simulink model "LQR_c_2017a"  (R2017a)
settings: Solver=VariableStepAuto  StartTime=0.0  StopTime=30  RelTol=1e-3
values from neighbouring files (symbols this model uses):
  LQRopt = lqrd(A,B,Q,R,8e-5)    [initParams.m]    (also in teste.m)
settings Model: Creator=seumagal  LastModifiedBy=seumagal

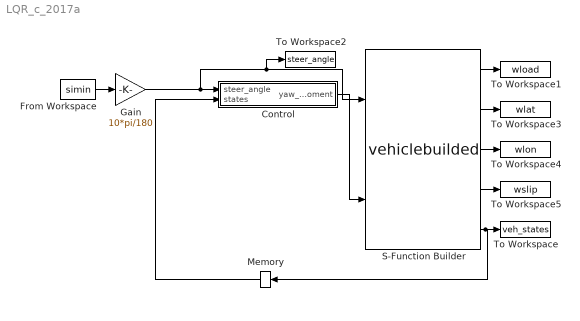
== system LQR_c_2017a ==
  "Control " : Subsystem  TreatAsAtomicUnit=on
  From Workspace : FromWorkspace  VariableName=simin  SampleTime=0
  Gain : Gain  Gain=10*pi/180
  Memory : Memory
  S-Function Builder : S-Function  InitFcn=try, set_param(gcb,'FunctionName','vehiclebuilded'), end  FunctionName=vehiclebuilded  Parameters=params  SFunctionModules=vehiclebuilded_wrapper  SFunctionDeploymentMode=off  EnableBusSupport=off  mask(S-Function Builder){}
      mask help: Simulink:masks:SFunctionBuilder_MD
      mask init:
      | val = [[.9  0.75 0.75 1 1 .9 .9 1]',[1 1 0.75 0.75 .9 .9 1 .9]'];try , sys = get_param(gcb,'SfunBuilderFcnName');if isempty(sys), sys = get_param(gcb,'FunctionName'); end,catch, sys = get_param(gcb,'FunctionName'); end
      settings: CopyFcn=set_param(gcbh,'LinkStatus','none')  PreSaveFcn=try, set_param(gcb,'FunctionName','vehiclebuilded'), end  OpenFcn=sfunctionwizard(gcbh)
      mask Display:
      | plot(val(:,1),val(:,2))
      | disp(sys)
      | port_label('input',1,'inSteer')
      | port_label('input',2,'inMz')
      | port_label('output',1,'outFz')
      | port_label('output',2,'outFy')
      | port_label('output',3,'outFx')
      | port_label('output',4,'outSlip')
      | port_label('output',5,'outStates')
  To Workspace : ToWorkspace  VariableName=veh_states  SaveFormat=Timeseries  SampleTime=-1
  To Workspace1 : ToWorkspace  VariableName=wload  SaveFormat=Timeseries  SampleTime=-1
  To Workspace2 : ToWorkspace  VariableName=steer_angle  SaveFormat=Timeseries  SampleTime=-1
  To Workspace3 : ToWorkspace  VariableName=wlat  SaveFormat=Timeseries  SampleTime=-1
  To Workspace4 : ToWorkspace  VariableName=wlon  SaveFormat=Timeseries  SampleTime=-1
  To Workspace5 : ToWorkspace  VariableName=wslip  SaveFormat=Timeseries  SampleTime=-1
  wires:
  From Workspace/1 -> Gain/1
  Gain/1 -> To Workspace2/1, S-Function Builder/1, "Control "/1(steer_angle)
  "Control "/1(yaw_moment) -> S-Function Builder/2
  Memory/1 -> "Control "/2(states)
  S-Function Builder/5 -> Memory/1, To Workspace/1
  S-Function Builder/1 -> To Workspace1/1
  S-Function Builder/3 -> To Workspace4/1
  S-Function Builder/2 -> To Workspace3/1
  S-Function Builder/4 -> To Workspace5/1

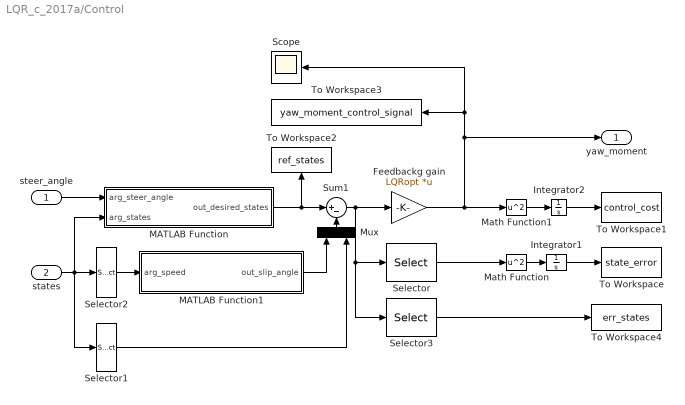
== system LQR_c_2017a/Control  ==
  steer_angle : Inport
  states : Inport  Port=2
  Feedbackg gain : Gain  Gain=LQRopt  Multiplication=Matrix(K*u)
  Integrator1 : Integrator
  Integrator2 : Integrator
  MATLAB Function : MATLAB Function  TreatAsAtomicUnit=on
  MATLAB Function1 : MATLAB Function  TreatAsAtomicUnit=on
  Math Function : Math  Operator=square  SaturateOnIntegerOverflow=on
  Math Function1 : Math  Operator=square  SaturateOnIntegerOverflow=on
  Mux : Mux  Inputs=2
  Scope : Scope
  Selector : Selector  InputPortWidth=4  IndexOptions=Index vector (dialog)  Indices=[1 2]  OutputSizes=1
  Selector1 : Selector  InputPortWidth=5  IndexOptions=Index vector (dialog)  Indices=[3,4,5]  OutputSizes=1
  Selector2 : Selector  InputPortWidth=5  IndexOptions=Index vector (dialog)  Indices=[1,2]  OutputSizes=1
  Selector3 : Selector  InputPortWidth=4  IndexOptions=Index vector (dialog)  Indices=[1 2]  OutputSizes=1
  Sum1 : Sum  Inputs=|+-
  To Workspace : ToWorkspace  VariableName=state_error  SaveFormat=Timeseries  SampleTime=-1
      settings: MaxDataPoints=1
  To Workspace1 : ToWorkspace  VariableName=control_cost  SaveFormat=Timeseries  SampleTime=-1
      settings: MaxDataPoints=1
  To Workspace2 : ToWorkspace  VariableName=ref_states  SaveFormat=Timeseries  SampleTime=-1
      settings: MaxDataPoints=Inf
  To Workspace3 : ToWorkspace  VariableName=yaw_moment_control_signal  SaveFormat=Timeseries  SampleTime=-1
      settings: MaxDataPoints=Inf
  To Workspace4 : ToWorkspace  VariableName=err_states  SaveFormat=Timeseries  SampleTime=-1
      settings: MaxDataPoints=Inf
  yaw_moment : Outport
  wires:
  Feedbackg gain/1 -> To Workspace3/1, Scope/1, yaw_moment/1, Math Function1/1
  steer_angle/1 -> MATLAB Function/1(arg_steer_angle)
  Math Function/1 -> Integrator1/1
  Integrator1/1 -> To Workspace/1
  Math Function1/1 -> Integrator2/1
  Integrator2/1 -> To Workspace1/1
  Selector/1 -> Math Function/1
  MATLAB Function/1(out_desired_states) -> Sum1/1, To Workspace2/1
  states/1 -> MATLAB Function/2(arg_states), Selector1/1, Selector2/1
  MATLAB Function1/1(out_slip_angle) -> Mux/1
  Selector2/1 -> MATLAB Function1/1(arg_speed)
  Mux/1 -> Sum1/2
  Selector1/1 -> Mux/2
  Sum1/1 -> Selector3/1, Selector/1, Feedbackg gain/1
  Selector3/1 -> To Workspace4/1

== matlab function LQR_c_2017a/Control /MATLAB Function1 ==
  data: arg_speed input; out_slip_angle output
function out_slip_angle = slipangle(arg_speed)

out_slip_angle = atan2(arg_speed(1),arg_speed(2));

== matlab function LQR_c_2017a/Control /MATLAB Function ==
  data: arg_steer_angle input; out_desired_states output; arg_states input
function  out_desired_states  = desired_states( arg_steer_angle, arg_states )

persistent mu_g;
persistent Ku;
persistent l;
if isempty(Ku)
    modelParams = coder.load( 'modelParam.mat' );
    Ku = modelParams.Ku;
    mu_g = modelParams.friction_coefficient*modelParams.g;
    l = modelParams.l;
end

long_speed = arg_states(2);
desired_yaw_rate =  long_speed*arg_steer_angle/(l + Ku*long_speed.^2);
max_yaw_rate = abs(mu_g/long_speed);

if abs(desired_yaw_rate) > max_yaw_rate
    desired_yaw_rate = max_yaw_rate*sign(desired_yaw_rate);
end
    
out_desired_states = [0; desired_yaw_rate; 0; 0 ];

end
